simulink model "ppg_whole2"  (R2020b)
settings: Solver=VariableStepAuto  StartTime=0.0  StopTime=10  RelTol=1e-3
libraries: fl_lib x28, nesl_utility x8, ee_lib x8
settings Model: Creator=Miodrag Bolic  LastModifiedBy=bolic
settings DataIOCC: ReturnWorkspaceOutputs=off
settings DebuggingCC: ArithmeticOperatorsInVariantConditions=warning
settings SFSimCC: CustomCodeUndefinedFunction=UseInterfaceOnly

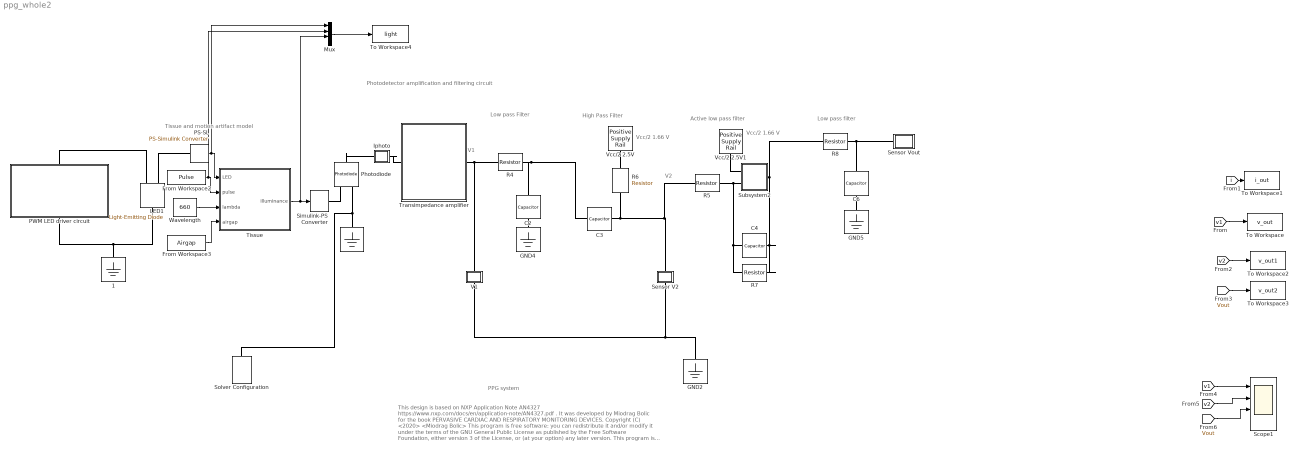
== system ppg_whole2 ==
  note: V1
  note: Low pass filter
  note: Active low pass filter
  note: High Pass Filter
  note: Low pass Filter
  note: V2
  note: Vcc/2
      | 1.66 V
  note: PPG system
  note: This design is based on NXP Application Note AN4327 https://www.nxp.com/docs/en/application-note/AN4327.pdf . It was developed by Miodrag Bolic for the book
      | PERVASIVE CARDIAC AND RESPIRATORY MONITORING DEVICES.
      |
      | Copyright (C) <2020> <Miodrag Bolic>
      | This program is free software: you can redistribute it and/or modify it under the terms of the GNU General Public License as published by the Free Software Foundation, either version 3 of the License, or (at your option) any later version. This program is distributed in the hope that it will be useful, but WITHOUT ANY WARRANTY; without even the implied warranty of MERCHANTABILITY or FITNESS FOR A PARTICULAR PURPOSE. See the GNU General Public License for more details <https://www.gnu.org/licenses/>.
  note: Tissue and motion artifact model
  note: Photodetector amplification and filtering circuit
  note: Vcc/2
      | 1.66 V
  " " : fl_lib/Electrical/Electrical Elements/Electrical Reference
  " 1" : fl_lib/Electrical/Electrical Elements/Electrical Reference
  C2 : fl_lib/Electrical/Electrical Elements/Capacitor  c=3.3 uF  r=1e-6 Ohm  g=0 1/Ohm  i_specify=off  i_priority=None  i=0 A  i_nominal_specify=off  i_nominal_unit=A  i_nominal_value=1  v_specify=off  v_priority=None  v=0 V  v_nominal_specify=off  v_nominal_unit=V  v_nominal_value=1  vc_specify=off  vc_priority=High  vc=0 V  vc_nominal_specify=off  vc_nominal_unit=V  vc_nominal_value=1
      settings: AttributesFormatString=%<c> %<c_unit>
  C3 : fl_lib/Electrical/Electrical Elements/Capacitor  c=3.3 uF  r=1e-6 Ohm  g=0 1/Ohm  i_specify=off  i_priority=None  i=0 A  i_nominal_specify=off  i_nominal_unit=A  i_nominal_value=1  v_specify=off  v_priority=None  v=0 V  v_nominal_specify=off  v_nominal_unit=V  v_nominal_value=1  vc_specify=off  vc_priority=High  vc=0 V  vc_nominal_specify=off  vc_nominal_unit=V  vc_nominal_value=1
      settings: AttributesFormatString=%<c> %<c_unit>
  C4 : fl_lib/Electrical/Electrical Elements/Capacitor  c=0.6 nF  r=1e-6 Ohm  g=0 1/Ohm  i_specify=off  i_priority=None  i=0 A  i_nominal_specify=off  i_nominal_unit=A  i_nominal_value=1  v_specify=off  v_priority=None  v=0 V  v_nominal_specify=off  v_nominal_unit=V  v_nominal_value=1  vc_specify=off  vc_priority=High  vc=0 V  vc_nominal_specify=off  vc_nominal_unit=V  vc_nominal_value=1
      settings: AttributesFormatString=%<c> %<c_unit>
  C6 : fl_lib/Electrical/Electrical Elements/Capacitor  c=1 uF  r=1e-6 Ohm  g=0 1/Ohm  i_specify=off  i_priority=None  i=0 A  i_nominal_specify=off  i_nominal_unit=A  i_nominal_value=1  v_specify=off  v_priority=None  v=0 V  v_nominal_specify=off  v_nominal_unit=V  v_nominal_value=1  vc_specify=off  vc_priority=High  vc=0 V  vc_nominal_specify=off  vc_nominal_unit=V  vc_nominal_value=1
      settings: AttributesFormatString=%<c> %<c_unit>
  From Workspace2 : FromWorkspace  VariableName=Pulse  SampleTime=0.0001  OutputAfterFinalValue=Setting to zero
  From Workspace3 : FromWorkspace  VariableName=Airgap  SampleTime=0.0001  OutputAfterFinalValue=Setting to zero
  GND2 : fl_lib/Electrical/Electrical Elements/Electrical Reference
  GND4 : fl_lib/Electrical/Electrical Elements/Electrical Reference
      settings: AttributesFormatString=\n
  GND5 : fl_lib/Electrical/Electrical Elements/Electrical Reference
  Iphoto : Subsystem
      mask Display: disp('i')
  LED1 : ee_lib/Sensors & Transducers/Light-Emitting Diode  Gain=0.05 W/A  prmExp=1  I12=[.0017, .003] A  V12=[.9, 1.05] V  IS=5e-5 A  ec=10  RS=0.1 Ohm  Tmeas=25 degC  C_param=1  CJ=20 pF  CJ0=20 pF  VJ=1 V  Mgrad=0.5  Vvec=[.1, 10, 100] V  Cvec=[15, 10, 2] pF  FC=0.5  T_param=1  IS_T2=1.8e-4 A  I1_T2=0.0034 A  V1_T2=1.05 V  Tmeas2=125 degC  EG_param=1  EG=1.11 eV  XTI_param=1  XTI=3  Tdevice=25 degC  i_capacitor_specify=off  i_capacitor_priority=High  i_capacitor=0 A  i_capacitor_nominal_specify=off  i_capacitor_nominal_unit=A  i_capacitor_nominal_value=1  v_capacitor_specify=off  v_capacitor_priority=None  v_capacitor=0 V  v_capacitor_nominal_specify=off  v_capacitor_nominal_unit=V  v_capacitor_nominal_value=1  thermal_network_parameterization=ee.enum.thermalNetworkTopology.cauer  Rth=[0, 10] K/W  Rth_Foster=[4, 6] K/W  thermal_mass_parameterization=ee.enum.thermalNetwork.timeconstant  thermal_mass=[0, 1] J/K  thermal_mass_Foster=[1.5, 3] J/K  thermal_time_constant=[0, 10] s  thermal_time_constant_Foster=[6, 18] s  thermal_mass_initial_temperatures=[25, 25] degC
      settings: SourceProductBaseCode=PS  InternalSimscapePortConfiguration="{\"Bottom\":[],\"Left\":[{\"id\":\"W\",\"label\":\"W\",\"type\":\"output\"},{\"id\":\"p\",\"label\":\"\",\"type\":\"foundation.electrical.electrical\"}],\"Right\":[{\"id\":\"n\",\"label\":\"\",\"type\":\"foundation.electrical.electrical\"}],\"Top\":[]}"
  Mux : Mux
  PS-SL : nesl_utility/PS-Simulink Converter  PhysicalDomain=network_engine_domain  SubClassName=ps_output  LeftPortType=input  RightPortType=output  PseudoPeriodic=off  Frequencies=[]  Unit=1  AffineConversion=off
  PWM LED driver circuit : Subsystem
      mask Display:
      | %plot([])
      | image('PWM1.png')
  Photodiode : ee_lib/Sensors & Transducers/Photodiode  prmFlux=1  Imeas=10 uA  FluxD=10 W/m^2  G=5e-6 m^2*A/W  prmExp=2  I2=0.1 A  V2=1.3 V  IS=5e-9 A  ec=3  RS=0.001 Ohm  Tmeas=25 degC  C_param=1  CJ=70 pF  CJ0=70 pF  VJ=1 V  Mgrad=0.5  Vvec=[ 0.1 10 100 ] V  Cvec=[ 45 30 6 ] pF  FC=0.5  T_param=1  IS_T2=2.5e-7 A  I1_T2=0.07000000000000001 A  V1_T2=1.3 V  Tmeas2=125 degC  EG_param=1  EG=1.11 eV  XTI_param=1  XTI=3  Tdevice=25 degC  i_capacitor_specify=off  i_capacitor_priority=High  i_capacitor=0 A  i_capacitor_nominal_specify=off  i_capacitor_nominal_unit=A  i_capacitor_nominal_value=1  v_capacitor_specify=off  v_capacitor_priority=None  v_capacitor=0 V  v_capacitor_nominal_specify=off  v_capacitor_nominal_unit=V  v_capacitor_nominal_value=1  thermal_network_parameterization=ee.enum.thermalNetworkTopology.cauer  Rth=[0, 10] K/W  Rth_Foster=[4, 6] K/W  thermal_mass_parameterization=ee.enum.thermalNetwork.timeconstant  thermal_mass=[0, 1] J/K  thermal_mass_Foster=[1.5, 3] J/K  thermal_time_constant=[0, 10] s  thermal_time_constant_Foster=[6, 18] s  thermal_mass_initial_temperatures=[25, 25] degC
      settings: SourceProductBaseCode=PS  InternalSimscapePortConfiguration="{\"Bottom\":[],\"Left\":[{\"id\":\"W\",\"label\":\"W\",\"type\":\"input\"},{\"id\":\"p\",\"label\":\"\",\"type\":\"foundation.electrical.electrical\"}],\"Right\":[{\"id\":\"n\",\"label\":\"\",\"type\":\"foundation.electrical.electrical\"}],\"Top\":[]}"
  R4 : fl_lib/Electrical/Electrical Elements/Resistor  R=2.7 kOhm  i_specify=off  i_priority=None  i=0 A  i_nominal_specify=off  i_nominal_unit=A  i_nominal_value=1  v_specify=off  v_priority=None  v=0 V  v_nominal_specify=off  v_nominal_unit=V  v_nominal_value=1
      settings: AttributesFormatString=%<R> %<R_unit>
  R5 : fl_lib/Electrical/Electrical Elements/Resistor  R=150 kOhm  i_specify=off  i_priority=None  i=0 A  i_nominal_specify=off  i_nominal_unit=A  i_nominal_value=1  v_specify=off  v_priority=None  v=0 V  v_nominal_specify=off  v_nominal_unit=V  v_nominal_value=1
      settings: AttributesFormatString=%<R> %<R_unit>
  R6 : fl_lib/Electrical/Electrical Elements/Resistor  R=280 kOhm  i_specify=off  i_priority=None  i=0 A  i_nominal_specify=off  i_nominal_unit=A  i_nominal_value=1  v_specify=off  v_priority=None  v=0 V  v_nominal_specify=off  v_nominal_unit=V  v_nominal_value=1
      settings: AttributesFormatString=%<R> %<R_unit>
  R7 : fl_lib/Electrical/Electrical Elements/Resistor  R=15 MOhm  i_specify=off  i_priority=None  i=0 A  i_nominal_specify=off  i_nominal_unit=A  i_nominal_value=1  v_specify=off  v_priority=None  v=0 V  v_nominal_specify=off  v_nominal_unit=V  v_nominal_value=1
      settings: AttributesFormatString=%<R> %<R_unit>
  R8 : fl_lib/Electrical/Electrical Elements/Resistor  R=3.3 kOhm  i_specify=off  i_priority=None  i=0 A  i_nominal_specify=off  i_nominal_unit=A  i_nominal_value=1  v_specify=off  v_priority=None  v=0 V  v_nominal_specify=off  v_nominal_unit=V  v_nominal_value=1
      settings: AttributesFormatString=%<R> %<R_unit>
  Scope1 : Scope  NumInputPorts=4
  Sensor V2 : Subsystem
      mask Display: disp('v')
  Sensor Vout : Subsystem
      mask Display: disp('Vo')
  Simulink-PS Converter : nesl_utility/Simulink-PS Converter  PhysicalDomain=network_engine_domain  SubClassName=ps_input  LeftPortType=input  RightPortType=output  PseudoPeriodic=off  Frequencies=[]  NoiseDistribution=none  NoiseParameters=[]  Unit=1  AffineConversion=off  FilteringAndDerivatives=zero  SimscapeFilterOrder=1  InputFilterTimeConstant=0.001  UdotUserProvided=1
  Solver Configuration : nesl_utility/Solver Configuration  PhysicalDomain=network_engine_domain  SubClassName=solver  LeftPortType=input  RightPortType=generic  Tones=[]  Harmonics=[]  SimulateNoise=off  Profile=off  UseLocalSampling=off  EnableSwitchedLinearOptims=on  FrequencyDomain=off  UseCCode=off  RelTol=0.001  AbsTol=1e-06  MinStep=1e-09  ToWorkspace=off  RevertToSquareIcSolve=off  NumHomotopyIterations=100  PhasorMode=off  PhasorModeNumHarmonics=1  DoDC=off  ResidualTolerance=1e-09  UseLocalSolver=off  LocalSolverChoice=NE_TRAPEZOIDAL_ADVANCER  LocalSolverSampleTime=0.000001  DoFixedCost=off  MaxNonlinIter=3  MaxModeIter=2  ComputeImpulses=off  ImpulseIterations=2  LinearAlgebra=Sparse  EquationFormulation=NE_TIME_EF  DelaysMemoryBudget=1024  AutomaticFiltering=on  FilteringTimeConstant=0.0001  PartitionStorageMethod=AS_NEEDED  PartitionMemoryBudget=1024  PartitionMethod=FAST
  Subsystem2 : Subsystem
      mask Display: image('op_amp_plus_up.png')
  Tissue : MATLAB Function  TreatAsAtomicUnit=on
  To Workspace : ToWorkspace  VariableName=v_out  SaveFormat=Timeseries  SampleTime=-1
  To Workspace1 : ToWorkspace  VariableName=i_out  SaveFormat=Timeseries  SampleTime=-1
  To Workspace2 : ToWorkspace  VariableName=v_out1  SaveFormat=Timeseries  SampleTime=-1
  To Workspace3 : ToWorkspace  VariableName=v_out2  SaveFormat=Timeseries  SampleTime=-1
  To Workspace4 : ToWorkspace  VariableName=light  SaveFormat=Timeseries  SampleTime=-1
  Transimpedance amplifier : Subsystem
      mask Display: image('Transimp1.png')
  V1 : Subsystem
      mask Display: disp('v')
  Vcc/2 2.5V : ee_lib/Sources/Positive Supply Rail  v0=1.66 V
      settings: SourceProductBaseCode=PS  InternalSimscapePortConfiguration="{\"Bottom\":[],\"Left\":[],\"Right\":[{\"id\":\"p\",\"label\":\"\",\"type\":\"foundation.electrical.electrical\"}],\"Top\":[]}"
  Vcc/2 2.5V1 : ee_lib/Sources/Positive Supply Rail  v0=1.66 V
      settings: SourceProductBaseCode=PS  InternalSimscapePortConfiguration="{\"Bottom\":[],\"Left\":[],\"Right\":[{\"id\":\"p\",\"label\":\"\",\"type\":\"foundation.electrical.electrical\"}],\"Top\":[]}"
  Wavelength : Constant  Value=660  SampleTime=0.0001
  wires:
  [v1] -> To Workspace/1
  [i] -> To Workspace1/1
  [v2] -> To Workspace2/1
  [Vout] -> To Workspace3/1
  Wavelength/1 -> Tissue/3(lambda)
  PS-SL/1 -> Mux/1, Tissue/1(LED)
  From Workspace3/1 -> Tissue/4(airgap)
  [v1] -> Scope1/1
  [v2] -> Scope1/2
  [Vout] -> Scope1/3
  Mux/1 -> To Workspace4/1
  From Workspace2/1 -> Mux/2, Tissue/2(pulse)
  Tissue/1(Illuminance) -> Mux/3, Simulink-PS Converter/1
  connections:
  Photodiode/LConn1 -- Simulink-PS Converter/RConn1
  Photodiode/RConn1 -- Iphoto/RConn1
  GND2/LConn1 -- Sensor V2/LConn1 -- V1/LConn1
  R4/RConn1 -- C3/LConn1 -- C2/LConn1
  C2/RConn1 -- GND4/LConn1
  Vcc/2 2.5V/RConn1 -- R6/LConn1
  Vcc/2 2.5V1/RConn1 -- Subsystem2/LConn1
  C3/RConn1 -- R6/RConn1 -- Sensor V2/RConn1 -- R5/LConn1
  R7/RConn1 -- C4/LConn1 -- R8/LConn1 -- Subsystem2/RConn1
  R7/LConn1 -- C4/RConn1 -- Subsystem2/LConn2 -- R5/RConn1
  GND5/LConn1 -- C6/RConn1
  R8/RConn1 -- Sensor Vout/LConn1 -- C6/LConn1
  LED1/LConn1 -- PS-SL/LConn1
  PWM LED driver circuit/LConn1 -- LED1/LConn2
  " "/LConn1 -- Photodiode/LConn2 -- Solver Configuration/RConn1
  R4/LConn1 -- V1/RConn1 -- Transimpedance amplifier/RConn1
  Iphoto/LConn1 -- Transimpedance amplifier/LConn1
  LED1/RConn1 -- " 1"/LConn1 -- PWM LED driver circuit/RConn1

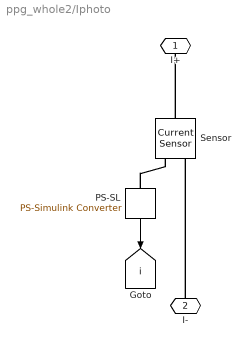
== system ppg_whole2/Iphoto ==
  PS-SL : nesl_utility/PS-Simulink Converter  PhysicalDomain=network_engine_domain  SubClassName=ps_output  LeftPortType=input  RightPortType=output  PseudoPeriodic=off  Frequencies=[]  Unit=1  AffineConversion=off
  Sensor : fl_lib/Electrical/Electrical Sensors/Current Sensor
      settings: SourceProductName=Foundation Library
  I+ : PMIOPort  Side=Right
  I- : PMIOPort  Port=2  Side=Left
  tag scope: i=global
  wires:
  PS-SL/1 -> [i]
  connections:
  PS-SL/LConn1 -- Sensor/RConn1
  Sensor/LConn1 -- I+/RConn1
  I-/RConn1 -- Sensor/RConn2

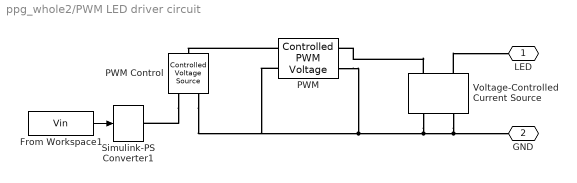
== system ppg_whole2/PWM LED driver circuit ==
  From Workspace1 : FromWorkspace  VariableName=Vin  SampleTime=0.0001  OutputAfterFinalValue=Setting to zero
  PWM : ee_lib/Integrated Circuits/Controlled PWM Voltage  F=1000 Hz  TD=0.3 ms  pulse_width_offset=0 s  pulse_min=0 s  Vmin=0 V  Vmax=5 V  Vm=3.3 V  pwm_or_av=1  event_type=1  sample_time=1e-6 s  u_min=0  u_max=1
  PWM Control : fl_lib/Electrical/Electrical Sources/Controlled Voltage Source
  Simulink-PS Converter1 : nesl_utility/Simulink-PS Converter  PhysicalDomain=network_engine_domain  SubClassName=ps_input  LeftPortType=input  RightPortType=output  PseudoPeriodic=off  Frequencies=[]  NoiseDistribution=none  NoiseParameters=[]  Unit=1  AffineConversion=off  FilteringAndDerivatives=zero  SimscapeFilterOrder=1  InputFilterTimeConstant=0.001  UdotUserProvided=1
  "Voltage-Controlled Current Source " : fl_lib/Electrical/Electrical Sources/Voltage-Controlled Current Source  K=0.005 1/Ohm  v1_specify=off  v1_priority=None  v1=0 V  v1_nominal_specify=off  v1_nominal_unit=V  v1_nominal_value=1  i2_specify=off  i2_priority=None  i2=0 A  i2_nominal_specify=off  i2_nominal_unit=A  i2_nominal_value=1
      settings: SourceProductBaseCode=SS  InternalSimscapePortConfiguration="{\"Bottom\":[],\"Left\":[{\"id\":\"p1\",\"label\":\"+\",\"type\":\"foundation.electrical.electrical\"},{\"id\":\"head\",\"label\":\"\",\"type\":\"foundation.electrical.electrical\"}],\"Right\":[{\"id\":\"n1\",\"label\":\"-\",\"type\":\"foundation.electrical.electrical\"},{\"id\":\"tail\",\"label\":\"\",\"type\":\"foundation.electrical.electrical\"}],\"Top\":[]}"
  LED : PMIOPort  Side=Left
  GND : PMIOPort  Port=2  Side=Right
  wires:
  From Workspace1/1 -> Simulink-PS Converter1/1
  connections:
  PWM Control/RConn2 -- PWM/LConn2 -- PWM/RConn2 -- "Voltage-Controlled Current Source "/RConn1 -- GND/RConn1 -- "Voltage-Controlled Current Source "/RConn2
  PWM/LConn1 -- PWM Control/LConn1
  PWM Control/RConn1 -- Simulink-PS Converter1/RConn1
  "Voltage-Controlled Current Source "/LConn1 -- PWM/RConn1
  "Voltage-Controlled Current Source "/LConn2 -- LED/RConn1

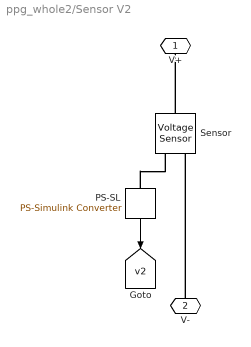
== system ppg_whole2/Sensor V2 ==
  PS-SL : nesl_utility/PS-Simulink Converter  PhysicalDomain=network_engine_domain  SubClassName=ps_output  LeftPortType=input  RightPortType=output  PseudoPeriodic=off  Frequencies=[]  Unit=1  AffineConversion=off
  Sensor : fl_lib/Electrical/Electrical Sensors/Voltage Sensor
      settings: SourceProductName=Foundation Library
  V+ : PMIOPort  Side=Right
  V- : PMIOPort  Port=2  Side=Left
  tag scope: v2=global
  wires:
  PS-SL/1 -> [v2]
  connections:
  PS-SL/LConn1 -- Sensor/RConn1
  Sensor/LConn1 -- V+/RConn1
  V-/RConn1 -- Sensor/RConn2

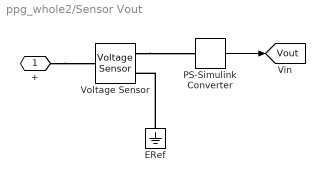
== system ppg_whole2/Sensor Vout ==
  ERef : fl_lib/Electrical/Electrical Elements/Electrical Reference
      settings: SourceProductName=Foundation Library
  PS-Simulink Converter : nesl_utility/PS-Simulink Converter  PhysicalDomain=network_engine_domain  SubClassName=ps_output  LeftPortType=input  RightPortType=output  PseudoPeriodic=off  Frequencies=[]  Unit=1  AffineConversion=off
      settings: SourceProductName=Utilities
  Voltage Sensor : fl_lib/Electrical/Electrical Sensors/Voltage Sensor
      settings: SourceProductName=Foundation Library
  + : PMIOPort  Side=Left
  tag scope: Vout=global
  wires:
  PS-Simulink Converter/1 -> [Vout]
  connections:
  ERef/LConn1 -- Voltage Sensor/RConn2
  Voltage Sensor/RConn1 -- PS-Simulink Converter/LConn1
  +/RConn1 -- Voltage Sensor/LConn1

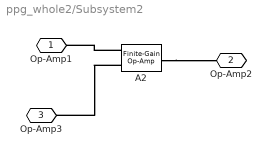
== system ppg_whole2/Subsystem2 ==
  A2 : ee_lib/Integrated Circuits/Finite-Gain Op-Amp  A=4.7e6  Rin=1e+6 Ohm  Rout=100 Ohm  Vmin=0 V  Vmax=3.3 V  noise_mode=0  v_noise=30e-9 V/Hz^0.50000  noise_prm=1  i_noise=0.5e-12 A/Hz^0.50000  ip_noise=0.5e-12 A/Hz^0.50000  in_noise=0.5e-12 A/Hz^0.50000  sample_time=1e-3 s  repeatability=1  auto_seed_v=2372152719  auto_seed_ip=936769862  auto_seed_in=3317287628  user_seed_v=0  user_seed_ip=0  user_seed_in=0
      settings: SourceProductBaseCode=PS  InternalSimscapePortConfiguration="{\"Bottom\":[],\"Left\":[{\"id\":\"p\",\"label\":\"+\",\"type\":\"foundation.electrical.electrical\"},{\"id\":\"n\",\"label\":\"-\",\"type\":\"foundation.electrical.electrical\"}],\"Right\":[{\"id\":\"out\",\"label\":\"\",\"type\":\"foundation.electrical.electrical\"}],\"Top\":[]}"
  Op-Amp1 : PMIOPort  Side=Left
  Op-Amp2 : PMIOPort  Port=2  Side=Right
  Op-Amp3 : PMIOPort  Port=3  Side=Left
  connections:
  A2/LConn1 -- Op-Amp1/RConn1
  A2/LConn2 -- Op-Amp3/RConn1
  A2/RConn1 -- Op-Amp2/RConn1

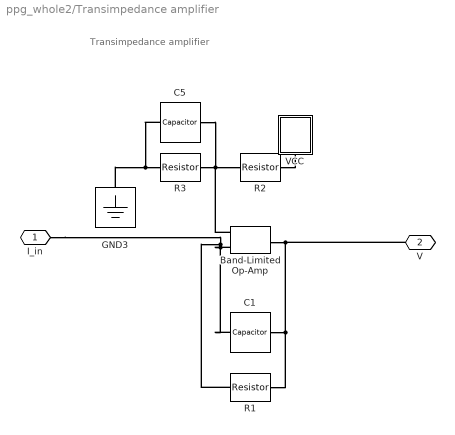
== system ppg_whole2/Transimpedance amplifier ==
  note: Transimpedance
      | amplifier
  Band-Limited Op-Amp : ee_lib/Integrated Circuits/Band-Limited Op-Amp  A=1000  Rin=1e8 Ohm  Rout=100 Ohm  Vmin=0 V  Vmax=3.3 V  Vdotmax=1000 V/s  f=1e5 Hz  V0=0 V
      settings: SourceProductBaseCode=PS
  C1 : fl_lib/Electrical/Electrical Elements/Capacitor  c=5 nF  r=1e-6 Ohm  g=0 1/Ohm  i_specify=off  i_priority=None  i=0 A  i_nominal_specify=off  i_nominal_unit=A  i_nominal_value=1  v_specify=off  v_priority=None  v=0 V  v_nominal_specify=off  v_nominal_unit=V  v_nominal_value=1  vc_specify=off  vc_priority=High  vc=0 V  vc_nominal_specify=off  vc_nominal_unit=V  vc_nominal_value=1
      settings: AttributesFormatString=|
      | %<c>
      | %<c_unit>
  C5 : fl_lib/Electrical/Electrical Elements/Capacitor  c=0.1 uF  r=1e-6 Ohm  g=0 1/Ohm  i_specify=off  i_priority=None  i=0 A  i_nominal_specify=off  i_nominal_unit=A  i_nominal_value=1  v_specify=off  v_priority=None  v=0 V  v_nominal_specify=off  v_nominal_unit=V  v_nominal_value=1  vc_specify=off  vc_priority=High  vc=0 V  vc_nominal_specify=off  vc_nominal_unit=V  vc_nominal_value=1
      settings: AttributesFormatString=|
      | %<c>
      | %<c_unit>
  GND3 : fl_lib/Electrical/Electrical Elements/Electrical Reference
      settings: AttributesFormatString=\n
  R1 : fl_lib/Electrical/Electrical Elements/Resistor  R=200 kOhm  i_specify=off  i_priority=None  i=0 A  i_nominal_specify=off  i_nominal_unit=A  i_nominal_value=1  v_specify=off  v_priority=None  v=0 V  v_nominal_specify=off  v_nominal_unit=V  v_nominal_value=1
      settings: AttributesFormatString=|
      | %<R>
      | %<R_unit>
  R2 : fl_lib/Electrical/Electrical Elements/Resistor  R=10 kOhm  i_specify=off  i_priority=None  i=0 A  i_nominal_specify=off  i_nominal_unit=A  i_nominal_value=1  v_specify=off  v_priority=None  v=0 V  v_nominal_specify=off  v_nominal_unit=V  v_nominal_value=1
      settings: AttributesFormatString=|
      | %<R>
      | %<R_unit>
  R3 : fl_lib/Electrical/Electrical Elements/Resistor  R=1.2 kOhm  i_specify=off  i_priority=None  i=0 A  i_nominal_specify=off  i_nominal_unit=A  i_nominal_value=1  v_specify=off  v_priority=None  v=0 V  v_nominal_specify=off  v_nominal_unit=V  v_nominal_value=1
      settings: AttributesFormatString=|
      | %<R>
      | %<R_unit>
  VCC : Subsystem
  I_in : PMIOPort  Side=Left
  V : PMIOPort  Port=2  Side=Right
  connections:
  R3/LConn1 -- Band-Limited Op-Amp/LConn1 -- C5/LConn1 -- R2/RConn1
  R1/LConn1 -- I_in/RConn1 -- C1/RConn1 -- Band-Limited Op-Amp/LConn2
  GND3/LConn1 -- C5/RConn1 -- R3/RConn1
  R2/LConn1 -- VCC/LConn1
  R1/RConn1 -- C1/LConn1 -- V/RConn1 -- Band-Limited Op-Amp/RConn1

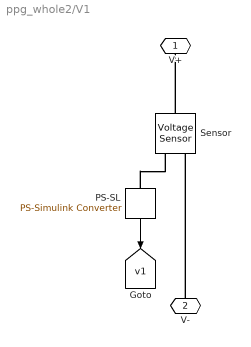
== system ppg_whole2/V1 ==
  PS-SL : nesl_utility/PS-Simulink Converter  PhysicalDomain=network_engine_domain  SubClassName=ps_output  LeftPortType=input  RightPortType=output  PseudoPeriodic=off  Frequencies=[]  Unit=1  AffineConversion=off
  Sensor : fl_lib/Electrical/Electrical Sensors/Voltage Sensor
      settings: SourceProductName=Foundation Library
  V+ : PMIOPort  Side=Right
  V- : PMIOPort  Port=2  Side=Left
  tag scope: v1=global
  wires:
  PS-SL/1 -> [v1]
  connections:
  PS-SL/LConn1 -- Sensor/RConn1
  Sensor/LConn1 -- V+/RConn1
  V-/RConn1 -- Sensor/RConn2

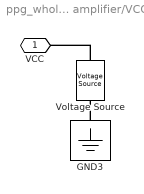
== system ppg_whole2/Transimpedance amplifier/VCC ==
  GND3 : fl_lib/Electrical/Electrical Elements/Electrical Reference
  Voltage Source : ee_lib/Sources/Voltage Source  dc_voltage=3.3 V  ac_voltage=0 V  ac_shift=0 rad  ac_frequency=0 Hz  noise_mode=0  PSD=0 V^2/Hz  repeatability=1  auto_seed=3621434445  user_seed=0  sample_time=1e-3 s  i_specify=off  i_priority=None  i=0 A  i_nominal_specify=off  i_nominal_unit=A  i_nominal_value=1  v_specify=off  v_priority=None  v=0 V  v_nominal_specify=off  v_nominal_unit=V  v_nominal_value=1
  VCC : PMIOPort  Side=Left
  connections:
  GND3/LConn1 -- Voltage Source/RConn1
  Voltage Source/LConn1 -- VCC/RConn1

== matlab function ppg_whole2/Tissue ==
  data: LED input double; pulse input double; lambda input double; Illuminance output double; airgap input

function Illuminance  = tissue(LED, pulse, lambda, airgap)
%global illum;
Illuminance  = zeros(1,1);
Illumination_Fraction=0.02;
if lambda == 660
    coef_lam=0.0002;
else
    coef_lam=0.00015;
end
Illuminance=LED*(Illum(lambda, airgap)-pulse*coef_lam)/(4e-6);



    
function Illumination_Fraction=  Illum(lambda, airgap)
    if lambda == 660
        Illumination_Fraction=5*(-9.83*airgap^2 +3.47*airgap+0.46)/100; %(8.7*airgap^2 +7.2*airgap+2.7)*0.01; 5 times is added to increase the illumination fraction
    else
        Illumination_Fraction=5*(-8.7*airgap^2 +2.18*airgap+0.77)/100; %(6.4*airgap^2 +5.4*airgap+2.3)*0.01;
    end
